simulink model "Demodulation_index_0_75"  (R2022b)
settings: Solver=VariableStepAuto  StartTime=0.0  StopTime=0.02  RelTol=1e-3
libraries: dspfdesign x1
settings Model: Creator=Sahaj Singh  LastModifiedBy=sahaj

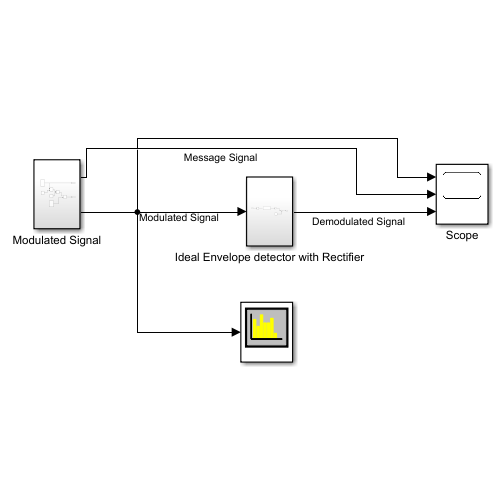
[thumbnail: Simulink's stored preview of the top-level diagram]
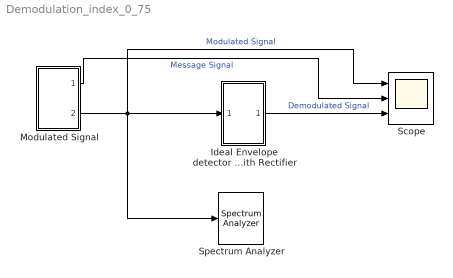
== system Demodulation_index_0_75 ==
  Ideal Envelope detector with Rectifier : Subsystem
  Modulated Signal : Subsystem
  Scope : Scope  NumInputPorts=3
  Spectrum Analyzer : SpectrumAnalyzer
  wires:
  Modulated Signal/2(" Modulated Signal Output") -> Spectrum Analyzer/1, Ideal Envelope detector with Rectifier/1(Modulated Signal), Scope/1  "Modulated Signal"
  Ideal Envelope detector with Rectifier/1(Demodualted Signal) -> Scope/3  "Demodulated Signal"
  Modulated Signal/1(Message Signal Output) -> Scope/2  "Message Signal"

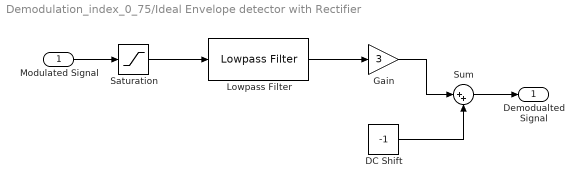
== system Demodulation_index_0_75/Ideal Envelope detector with Rectifier ==
  Modulated Signal : Inport
  DC Shift : Constant  Value=-1
  Gain : Gain  Gain=3
  Lowpass Filter : dspfdesign/Lowpass Filter  FilterType=FIR  DesignForMinimumOrder=on  FilterOrder=50  PassbandFrequency=4e3  StopbandFrequency=10e3  PassbandRipple=1  StopbandAttenuation=80  InheritSampleRate=off  SampleRate=500000  SimulateUsing=Interpreted execution  roundingMode=Floor  coeffsDataTypeStr=fixdt(1,16)
  Saturation : Saturate  UpperLimit=2  LowerLimit=0
  Sum : Sum  Inputs=|++
  Demodualted Signal : Outport
  wires:
  Saturation/1 -> Lowpass Filter/1
  Lowpass Filter/1 -> Gain/1
  Sum/1 -> Demodualted Signal/1
  Gain/1 -> Sum/1
  Modulated Signal/1 -> Saturation/1
  DC Shift/1 -> Sum/2

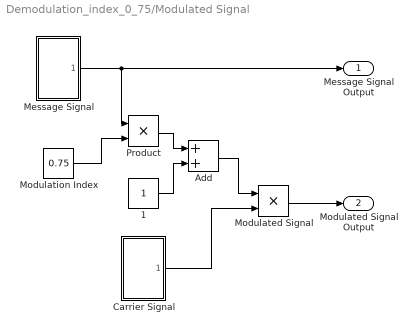
== system Demodulation_index_0_75/Modulated Signal ==
  1 : Constant
  Add : Sum
  Carrier Signal : Subsystem
  Message Signal : Subsystem
  Modulated Signal : Product
  Modulation Index : Constant  Value=0.75
  Product : Product
  Message Signal Output : Outport
  " Modulated Signal Output" : Outport  Port=2
  wires:
  Carrier Signal/1(Carrier Signal) -> Modulated Signal/2
  Message Signal/1(Message Signal) -> Product/1, Message Signal Output/1
  Modulated Signal/1 -> " Modulated Signal Output"/1
  Modulation Index/1 -> Product/2
  Product/1 -> Add/1
  1/1 -> Add/2
  Add/1 -> Modulated Signal/1

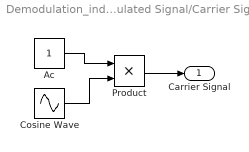
== system Demodulation_index_0_75/Modulated Signal/Carrier Signal ==
  Ac : Constant
  Cosine Wave : Sin  Frequency=125663.706137  Phase=-pi/2  SampleTime=0.000002
  Product : Product
  Carrier Signal : Outport
  wires:
  Ac/1 -> Product/1
  Cosine Wave/1 -> Product/2
  Product/1 -> Carrier Signal/1

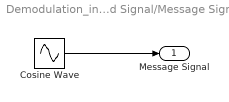
== system Demodulation_index_0_75/Modulated Signal/Message Signal ==
  Cosine Wave : Sin  Frequency=12566.370614  Phase=-pi/2  SampleTime=0.000002
  Message Signal : Outport
  wires:
  Cosine Wave/1 -> Message Signal/1
